simulink model "Example_12_3_2_2"  (R2018a)
settings: Solver=FixedStepAuto  StartTime=0.0  StopTime=10.0  FixedStep=0.001  RelTol=1e-3
settings Model: Creator=ahmed  LastModifiedBy=ahmed

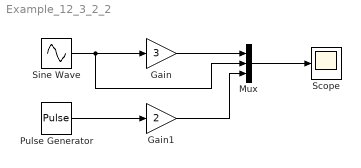
== system Example_12_3_2_2 ==
  Gain : Gain  Gain=3
  Gain1 : Gain  Gain=2
  Mux : Mux  Inputs=3
  Pulse Generator : DiscretePulseGenerator  PulseType=Time based  PulseWidth=50
  Scope : Scope
  Sine Wave : Sin  SampleTime=0
  wires:
  Gain/1 -> Mux/1
  Sine Wave/1 -> Mux/2, Gain/1
  Mux/1 -> Scope/1
  Pulse Generator/1 -> Gain1/1
  Gain1/1 -> Mux/3
